simulink model "signals2"  (R2019b)
settings: Solver=VariableStepAuto  StartTime=0.0  StopTime=inf  RelTol=1e-3  EnableMultiTasking=on
StartFcn:
  | %EventListener
  | h = add_exec_event_listener('signals2/signals Generator','PostOutputs',@EventListener);
libraries: sldrtlib x1, aerolibanimutils x1
settings Model: EnablePacing=on  Creator=zhan.xiong  LastModifiedBy=HUAWEI
settings DataIOCC: ReturnWorkspaceOutputs=off
settings OptimizationCC: LifeSpan=inf
settings DebuggingCC: SFUnexpectedBacktrackingDiag=warning  SFNoUnconditionalDefaultTransitionDiag=warning  ArithmeticOperatorsInVariantConditions=warning
settings SFSimCC: SimUseLocalCustomCode=off  CustomCodeUndefinedFunction=UseInterfaceOnly
settings RTWCC: RTWUseLocalCustomCode=off
settings CodeAppCC: StateflowObjectComments=on
settings GRTTargetCC: TargetLangStandard=C89/C90 (ANSI)  GeneratePreprocessorConditionals=Disable all
settings ConfigComp: CovMetricSettings=dw  CovHtmlReporting=on  CovSaveCumulativeToWorkspaceVar=on  CovSaveSingleToWorkspaceVar=on  CovExternalEMLEnable=off

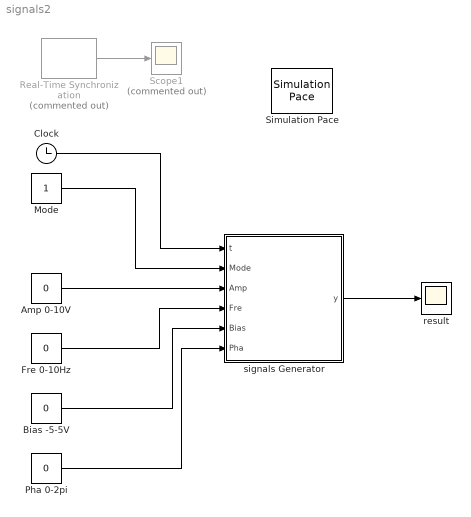
== system signals2 ==
  Amp 0-10V : Constant  Value=0  OutMin=[0]  OutMax=[10]
  Bias -5-5V : Constant  Value=0  OutMin=[-5]  OutMax=[5]
  Clock : Clock
  Fre 0-10Hz : Constant  Value=0  OutMin=[0]  OutMax=[10]
  Mode : Constant
  Pha 0-2pi : Constant  Value=0  OutMin=[0]  OutMax=[2*pi]
  Real-Time Synchronization : sldrtlib/Real-Time Synchronization  Commented=on  SampleTime=0.1  MaxMissedTicks=inf  ShowMissedTicks=on  YieldWhenWaiting=on
  Scope1 : Scope  Commented=on
  Simulation Pace : aerolibanimutils/Simulation Pace  SimulationPace=1  SleepMode=MATLAB Thread  OutputPaceError=off  SampleTime=1/30
  "result " : Scope
  signals Generator : MATLAB Function  TreatAsAtomicUnit=on
  wires:
  Real-Time Synchronization/1 -> Scope1/1
  Pha 0-2pi/1 -> signals Generator/6(Pha)
  signals Generator/1(y) -> "result "/1
  Amp 0-10V/1 -> signals Generator/3(Amp)
  Bias -5-5V/1 -> signals Generator/5(Bias)
  Mode/1 -> signals Generator/2(Mode)
  Clock/1 -> signals Generator/1(t)
  Fre 0-10Hz/1 -> signals Generator/4(Fre)

== matlab function signals2/signals Generator ==
  data: t input; y output; Mode input; Amp input; Fre input; Bias input; Pha input
% @discription: different types of signal generator function
% @Author：Zhang Yifan
% @date:2020-4-17 16:28
function y = fcn(t,Mode,Amp,Fre,Bias,Pha)
%产生周期性待调制的锯齿波 范围-pi至pi
temp = mod(2*pi*Fre*t+Pha,2*pi)-pi;
if Mode == 1
    y = Amp*sin(temp)+Bias;
elseif Mode == 2
    y = Amp*sign(sin(temp))+Bias;
elseif Mode == 3
    y = Amp*(abs(temp)-pi/2)/(pi/2)+Bias;
else
    y = 0;
end
